simulink model "Group31_ProjectWork_EmbeddedSystem"  (R2024b)
settings: Solver=FixedStepDiscrete  StartTime=0.0  StopTime=100  FixedStep=0.1  RelTol=1e-3  EnableMultiTasking=on
libraries: stm32f4xxblockslib x6, stm32g4xxblockslib x2, stm32blockslib x2
settings Model: STM32="{\"UARTRead\":[{\"ID\":\"ProgettoEmbedded_LI_ST_gruppo33_backup_2:87\"},{\"ID\":\"ProgettoEmbedded_LI_ST_gruppo33_backup_3:87\"},{\"ID\":\"ProgettoEmbedded_LI_ST_gruppo33:87\"},{\"ID\":\"Group31_ProjectWork_EmbeddedSystem:87\"}],\"UARTWrite\":[{\"ID\":\"ProgettoEmbedded_LI_ST_gruppo33_backup_2:92\"},{\"ID\":\"ProgettoEmbedded_LI_ST_gruppo33_backup_3:92\"},{\"ID\":\"ProgettoEmbedded_LI_ST_gruppo33:92\"},{\"ID\":\"Group31_ProjectWork_EmbeddedSystem:92\"}],\"PWMOutput\":[{\"ID\":\"ProgettoEmbedded_LI_ST_gruppo33_backup_2:88\"},{\"ID\":\"ProgettoEmbedded_LI_ST_gruppo33_backup_2:104\"},{\"ID\":\"ProgettoEmbedded_LI_ST_gruppo33_backup_3:104\"},{\"ID\":\"ProgettoEmbedded_LI_ST_gruppo33_backup_3:88\"},{\"ID\":\"ProgettoEmbedded_LI_ST_gruppo33:104\"},{\"ID\":\"ProgettoEmbedded_LI_ST_gruppo33:88\"},{\"ID\":\"Group31_ProjectWork_EmbeddedSystem:104\"},{\"ID\":\"Group31_ProjectWork_EmbeddedSystem:88\"}],\"DigitalPortRead\":[{\"ID\":\"ProgettoEmbedded_LI_ST_gruppo33_backup_2:83\"},{\"ID\":\"ProgettoEmbedded_LI_ST_gruppo33_backup_2:99\"},{\"ID\":\"ProgettoEmbedded_LI_ST_gruppo33_backup_2:100\"},{\"ID\":\"ProgettoEmbedded_LI_ST_gruppo33_backup_2:101\"},{\"ID\":\"ProgettoEmbedded_LI_ST_gruppo33_backup_3:101\"},{\"ID\":\"ProgettoEmbedded_LI_ST_gruppo33_backup_3:100\"},{\"ID\":\"ProgettoEmbedded_LI_ST_gruppo33_backup_3:99\"},{\"ID\":\"ProgettoEmbedded_LI_ST_gruppo33_backup_3:83\"},{\"ID\":\"ProgettoEmbedded_LI_ST_gruppo33:101\"},{\"ID\":\"ProgettoEmbedded_LI_ST_gruppo33:100\"},{\"ID\":\"ProgettoEmbedded_LI_ST_gruppo33:99\"},{\"ID\":\"ProgettoEmbedded_LI_ST_gruppo33:83\"},{\"ID\":\"Group31_ProjectWork_EmbeddedSystem:101\"},{\"ID\":\"Group31_ProjectWork_EmbeddedSystem:100\"},{\"ID\":\"Group31_ProjectWork_EmbeddedSystem:99\"},{\"ID\":\"Group31_ProjectWork_EmbeddedSystem:83\"}],\"DigitalPortWrite\":[{\"ID\":\"ProgettoEmbedded_LI_ST_gruppo33_backup_2:93\"},{\"ID\":\"ProgettoEmbedded_LI_ST_gruppo33_backup_2:105\"},{\"ID\":\"ProgettoEmbedded_LI_ST_gruppo33_backup_3:105\"},{\"ID\":\"ProgettoEmbedded_LI_ST_gruppo33_backup_3:93\"},{\"ID\":\"ProgettoEmbedded_LI_ST_gruppo33:105\"},{\"ID\":\"ProgettoEmbedded_LI_ST_gruppo33:93\"},{\"ID\":\"Group31_ProjectWork_EmbeddedSystem:105\"},{\"ID\":\"Group31_ProjectWork_EmbeddedSystem:93\"}]}"  PacingRate=0.400000  Creator=nancy  LastModifiedBy=Alessandro
settings SolverCC: AlgebraicLoopSolver=TrustRegion  AutoInsertRateTranBlk=on
settings DataIOCC: LimitDataPoints=on
settings OptimizationCC: DefaultParameterBehavior=Inlined  EnhancedBackFolding=on  PassReuseOutputArgsAs=Individual arguments  ZeroExternalMemoryAtStartup=off  ZeroInternalMemoryAtStartup=off  MaxStackSize=512  OptimizeBlockOrder=speed  DifferentSizesBufferReuse=on  OptimizationCustomize=off  EfficientTunableParamExpr=on
settings DebuggingCC: ParameterTunabilityLossMsg=error  UnconnectedInputMsg=warning  UnconnectedOutputMsg=warning  UnconnectedLineMsg=warning  AllowSymbolicDim=off  SFUnexpectedBacktrackingDiag=warning  SFNoUnconditionalDefaultTransitionDiag=warning  SFExecutionAtInitializationDiag=none  ArithmeticOperatorsInVariantConditions=warning
settings HardwareCC: ProdBitPerPointer=32  ProdBitPerSizeT=32  ProdBitPerPtrDiffT=32  ProdLargestAtomicInteger=Long  ProdLargestAtomicFloat=Double  ProdWordSize=32  ProdLongLongMode=on  ProdHWDeviceType=ARM Compatible->ARM Cortex-M
settings ModelReferenceCC: EnableRefExpFcnMdlSchedulingChecks=on
settings SFSimCC: SimUseLocalCustomCode=off  CustomCodeUndefinedFunction=UseInterfaceOnly
settings RTWCC: Description=Embedded Coder  SystemTargetFile=ert.tlc  HardwareBoard=STM32G4xx Based  TemplateMakefile=ert_default_tmf  RTWUseLocalCustomCode=off  Toolchain=GNU Tools for ARM Embedded Processors  GPUComputeCapability=3.5  DLArmComputeVersion=19.05
settings CodeAppCC: ForceParamTrailComments=on  IgnoreCustomStorageClasses=off  OperatorAnnotations=on  SimulinkDataObjDesc=on  SFDataObjDesc=on  InsertBlockDesc=on
settings ERTTargetCC: TargetLangStandard=C99 (ISO)  CodeReplacementLibrary=ARM Cortex-M  SupportVariableSizeSignals=on  ExtModeTransport=3  ExtModeStaticAlloc=on  ExtModeStaticAllocSize=2048  ExtModeMexFile=ext_xcp  ExtModeIntrfLevel=Level2 - Open
settings ConfigComp: CovMetricSettings=dw  CovSaveCumulativeToWorkspaceVar=on  CovSaveSingleToWorkspaceVar=on  CovExternalEMLEnable=off  CovSFcnEnable=off

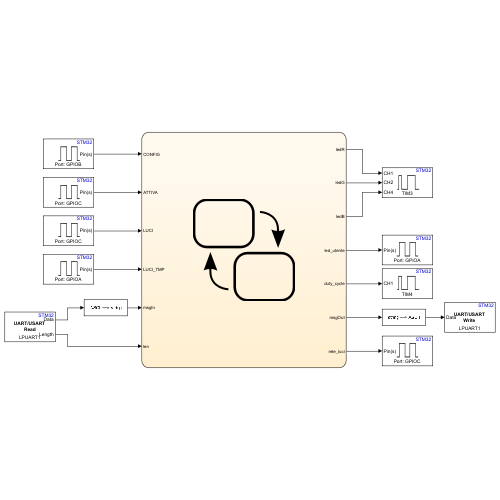
[thumbnail: Simulink's stored preview of the top-level diagram]
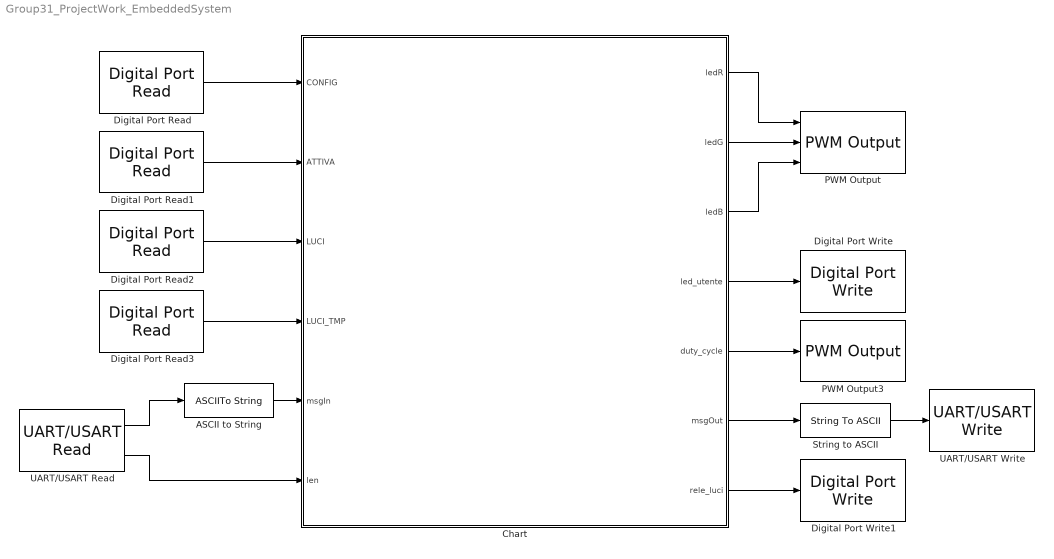
== system Group31_ProjectWork_EmbeddedSystem ==
  ASCII to String : ASCIIToString
  Chart : Stateflow chart  TreatAsAtomicUnit=on
  Digital Port Read : stm32f4xxblockslib/Digital Port Read  PortName=GPIOB  PinNumber=[0]  ReadOperation=on  IOAsArray=on  SampleTime=-1  EnableSimPort=off  hoistedMaskSrc=ECSoC/ECSimCodegen/Digital Port Read
      settings: LibrarySourceBlock=stm32g4xxblockslib/Digital Port Read
  Digital Port Read1 : stm32f4xxblockslib/Digital Port Read  PortName=GPIOC  PinNumber=[13]  ReadOperation=on  IOAsArray=on  SampleTime=-1  EnableSimPort=off  hoistedMaskSrc=ECSoC/ECSimCodegen/Digital Port Read
      settings: LibrarySourceBlock=stm32g4xxblockslib/Digital Port Read
  Digital Port Read2 : stm32f4xxblockslib/Digital Port Read  PortName=GPIOC  PinNumber=[10]  ReadOperation=on  IOAsArray=on  SampleTime=-1  EnableSimPort=off  hoistedMaskSrc=ECSoC/ECSimCodegen/Digital Port Read
      settings: LibrarySourceBlock=stm32g4xxblockslib/Digital Port Read
  Digital Port Read3 : stm32f4xxblockslib/Digital Port Read  PortName=GPIOA  PinNumber=[15]  ReadOperation=on  IOAsArray=on  SampleTime=-1  EnableSimPort=off  hoistedMaskSrc=ECSoC/ECSimCodegen/Digital Port Read
      settings: LibrarySourceBlock=stm32g4xxblockslib/Digital Port Read
  Digital Port Write : stm32f4xxblockslib/Digital Port Write  PortName=GPIOA  PinNumber=[5]  ReadOperation=off  IOAsArray=on  EnableSimPort=off  hoistedMaskSrc=ECSoC/ECSimCodegen/Digital Port Write
      settings: LibrarySourceBlock=stm32g4xxblockslib/Digital Port Write
  Digital Port Write1 : stm32f4xxblockslib/Digital Port Write  PortName=GPIOC  PinNumber=[2]  ReadOperation=off  IOAsArray=on  EnableSimPort=off  hoistedMaskSrc=ECSoC/ECSimCodegen/Digital Port Write
      settings: LibrarySourceBlock=stm32g4xxblockslib/Digital Port Write
  PWM Output : stm32g4xxblockslib/PWM Output  TimerModule=TIM3  DutycycleUnits=Percentage  EnableChannel1=on  EnableChannel2=on  EnableChannel3=off  EnableChannel4=on  EnableChannel5=off  EnableChannel6=off  EnableCounterInput=off  EnableMainOutputInput=off  EnableFrequencyInput=off  SetRCAfterCE=off  OutputDirection=off  OutputMainOutputEnableStatus=off  SampleTime=0.1  EnableSimPort=off  EnableUpdateEvent=off  EnableCaptureCompare1Event=off  EnableCaptureCompare2Event=off  EnableCaptureCompare3Event=off  EnableCaptureCompare4Event=off  EnableTriggerEvent=off  EnableBreakEvent=off  EnableBreakEvent2=off  ProcessorFamily=STM32G4  hoistedMaskSrc=ECSoC/ECSimCodegen/PWM Output
  PWM Output3 : stm32g4xxblockslib/PWM Output  TimerModule=TIM4  DutycycleUnits=Percentage  EnableChannel1=on  EnableChannel2=off  EnableChannel3=off  EnableChannel4=off  EnableChannel5=off  EnableChannel6=off  EnableCounterInput=off  EnableMainOutputInput=off  EnableFrequencyInput=off  SetRCAfterCE=off  OutputDirection=off  OutputMainOutputEnableStatus=off  SampleTime=0.1  EnableSimPort=off  EnableUpdateEvent=off  EnableCaptureCompare1Event=off  EnableCaptureCompare2Event=off  EnableCaptureCompare3Event=off  EnableCaptureCompare4Event=off  EnableTriggerEvent=off  EnableBreakEvent=off  EnableBreakEvent2=off  ProcessorFamily=STM32G4  hoistedMaskSrc=ECSoC/ECSimCodegen/PWM Output
  String to ASCII : StringToASCII  OutputVectorSize=127
  UART/USART Read : stm32blockslib/UART//USART Read  UARTModule=LPUART1  DataType=uint8  DataLength=1  BlockingMode=off  BlockingTimeout=0.1  OutputLength=on  OutputStatus=off  SampleTime=-1
      settings: LibrarySourceBlock=stm32g4xxblockslib/UART//USART Read
  UART/USART Write : stm32blockslib/UART//USART Write  UARTModule=LPUART1  LengthOfDataToSend=off  BlockingMode=off  BlockingTimeout=0.1  OutputStatus=off
      settings: LibrarySourceBlock=stm32g4xxblockslib/UART//USART Write
  wires:
  Chart/4(led_utente) -> Digital Port Write/1
  Digital Port Read/1 -> Chart/1(CONFIG)
  Chart/1(ledR) -> PWM Output/1
  Chart/6(msgOut) -> String to ASCII/1
  String to ASCII/1 -> UART/USART Write/1
  Digital Port Read1/1 -> Chart/2(ATTIVA)
  Digital Port Read2/1 -> Chart/3(LUCI)
  Digital Port Read3/1 -> Chart/4(LUCI_TMP)
  Chart/5(duty_cycle) -> PWM Output3/1
  Chart/7(rele_luci) -> Digital Port Write1/1
  Chart/2(ledG) -> PWM Output/2
  Chart/3(ledB) -> PWM Output/3
  UART/USART Read/2 -> Chart/6(len)
  UART/USART Read/1 -> ASCII to String/1
  ASCII to String/1 -> Chart/5(msgIn)

== stateflow chart Group31_ProjectWork_EmbeddedSystem/Chart ==
  state Group31_ProjectWork_EmbeddedSystem
    state INATTIVO
      en: msgOut = "Premere il pulsante ATTIVA per attivare il dispositivo" + char([13 10]) + char([13 10]);
      temperatura = 16; strTemperatura = "16";
      ledR = 0;  ledG = 0;  ledB = 255;
      led_utente = 0;
      rele_luci = 0;
      angolo = 0; strAngolo = "0";
      duty_cycle = 5;
      durata_luci = 0; strDurataLuci = "0";
      mod_luci = 0; strModLuci = "0";
      du: msgOut = "";
    state CLEAR
      en: msgOut = sprintf("\033[0;0H\033[2J");
    state ATTIVO
      state MAIN [parallel]
        settings: executionOrder=1
        state CONFIGURAZIONE
          ex:  prima_attivazione = 0;
          state CONFIGURAZIONE_COMPLETATA
            en: config_comp_init = 1;
            msgOut = char([13 10]) + fine_configurazione_iniziale();
            du: msgOut = "";
          state PRECONFIG
            en: msgOut = "";
          state INIT
            en: msgOut = initMenu();
            du: msgOut ="";
          state MENU
            en: msgOut = char([13 10]) + prepareMenu;
            du: msgOut = "";
          state setTemperatura
            en: msgOut = char([13 10]) + "TEMPERATURA: Range 16 C - 30 C" + char([13 10]);
            du: msgOut = "";
          state setVeneziane
            en: msgOut = char([13 10]) + "VENEZIANE: 0 - 9" + char([13 10]);
            du: msgOut = "";
          state setDurataLuci
            en: msgOut = char([13 10]) + "MODALITA LUCI TEMPORIZZATE: durata di accensione (5 - 30 s, 0 s: disattivata)" + char([13 10]);
            du: msgOut = "";
          state setModalitaLuci
            en: msgOut = char([13 10]) + "MODALITA LUCI: (0: spento, 1: acceso)" + char([13 10]);
            du: msgOut = "";
          state setTemperatura1
            en: uartMsg = uartMsg + msgIn;
            msgOut = msgIn; i = i + 1;
            if i == 2
            config_comp_temp = configTemperatura(uartMsg);
            end
            du: msgOut = "";
          state setVeneziane1
            en: uartMsg = uartMsg + msgIn;
            msgOut = msgIn;
            config_comp_ven = configVeneziane(uartMsg);
            du: msgOut = "";
          state setDurataLuci1
            en: uartMsg = uartMsg + msgIn;
            msgOut = msgIn; i = i + 1;
            if i > 0 && i < 3
            config_comp_durata_luci = configDurataLuci(uartMsg);
            end
            du: msgOut = "";
          state setModalitaLuci1
            en: uartMsg = uartMsg + msgIn; msgOut = msgIn;
            config_comp_mod_luci = configModLuci(uartMsg);
            du: msgOut = "";
          state ErrorDurataLuci
            en: msgOut = errorDurataLuci();
            du: msgOut = "";
          state ErrorTemperatura
            en: msgOut = errorTemperatura();
            du: msgOut = "";
          state ErrorVeneziane
            en: msgOut = errorVeneziane();
            du: msgOut = "";
          state ErrorModLuci
            en: msgOut = errorModLuci();
            du: msgOut = "";
          (default) -> PRECONFIG
          PRECONFIG -> INIT [order 2] : [prima_attivazione == 1]
          PRECONFIG -> MENU [order 1] : [prima_attivazione == 0]
          (junction 455) -> CONFIGURAZIONE_COMPLETATA [order 2] : [prima_attivazione == 1]
          (junction 455) -> MENU [order 1] : [prima_attivazione == 0]
          MENU -> setModalitaLuci [order 1] : [len > 0 && msgIn == "1"]
          MENU -> setVeneziane [order 3] : [len > 0 && msgIn == "4"]
          (junction 529) -> MENU [order 2] : {prima_attivazione == 0}
          (junction 430) -> MENU [order 1] : [prima_attivazione == 0]
          MENU -> setDurataLuci [order 4] : [len > 0 && msgIn == "2"]
          (junction 427) -> MENU [order 1] : [prima_attivazione == 0]
          MENU -> setTemperatura [order 2] : [len > 0 && msgIn == "3"]
          INIT -> setModalitaLuci : after(3,sec)
          (junction 529) -> setDurataLuci [order 1] : [prima_attivazione == 1]
          (junction 430) -> setVeneziane [order 2] : [prima_attivazione == 1]
          setVeneziane1 -> (junction 455) [order 1] : [config_comp_ven == 1 && len > 0 && msgIn == char(13)]{angolo = applyConv(uartMsg); strAngolo = uartMsg;}
          setVeneziane -> setVeneziane1 : [len >0]{uartMsg="";}
          ErrorVeneziane -> setVeneziane : [len > 0 && msgIn == char(13)]
          setDurataLuci -> setDurataLuci1 : [len >0]{uartMsg=""; i = 0;}
          ErrorDurataLuci -> setDurataLuci : [len > 0 && msgIn == char(13)]
          setModalitaLuci -> setModalitaLuci1 : [len > 0]{uartMsg="";}
          ErrorModLuci -> setModalitaLuci : [len > 0 && msgIn == char(13)]
          (junction 427) -> setTemperatura [order 2] : [prima_attivazione == 1]
          setTemperatura -> setTemperatura1 : [len >0]{uartMsg=""; i = 1;}
          ErrorTemperatura -> setTemperatura : [len > 0 && msgIn == char(13)]
          setModalitaLuci1 -> (junction 529) [order 1] : [config_comp_mod_luci == 1 && len > 0 && msgIn == char(13)]{mod_luci = applyConv(uartMsg); strModLuci = uartMsg;}
          setDurataLuci1 -> (junction 427) [order 1] : [config_comp_durata_luci == 1 && len > 0 && msgIn == char(13)]{durata_luci = applyConv(uartMsg); strDurataLuci = uartMsg;}
          setTemperatura1 -> (junction 430) [order 2] : [config_comp_temp == 1 && len > 0 && msgIn == char(13)]{temperatura = applyConv(uartMsg); strTemperatura = uartMsg;}
          setDurataLuci1 -> setDurataLuci1 [order 3] : [rising(len)]
          setTemperatura1 -> setTemperatura1 [order 3] : [rising(len)]
          setModalitaLuci1 -> ErrorModLuci [order 2] : [config_comp_mod_luci == 0 && len > 0 && msgIn == char(13)]
          setDurataLuci1 -> ErrorDurataLuci [order 2] : [config_comp_durata_luci == 0 && len > 0 && msgIn == char(13)]
          setTemperatura1 -> ErrorTemperatura [order 1] : [config_comp_temp == 0 && len > 0 && msgIn == char(13)]
          setVeneziane1 -> ErrorVeneziane [order 2] : [config_comp_ven == 0 && len > 0 && msgIn == char(13)]
        state OPERAZIONE
          state NOTIFICA_STATO [parallel]
            settings: executionOrder=2
            state NOT2
              en: %% VENEZIANE
              if angolo == 0
              printVen = "CHIUSE";
              elseif angolo == 9
              printVen = "APERTE";
              else
              printVen = "APERTE PARZIALMENTE con Preset " + strAngolo;
              end
              %% LUCI
              if rele_luci == 1 || mod_luci == 1
              printLuci = "ACCESE";
              else
              printLuci = "SPENTE";
              end
              msgOut =  char([13 10]) + notifica(strTemperatura, printVen, printLuci) + char([13 10]);
              du: msgOut = "";
            (default) -> NOT2
            NOT2 -> NOT2 : after(10, sec)
          state LUCI [parallel]
            settings: executionOrder=3
            state LUCI_SPENTE
              en: rele_luci = 0;
              mod_luci = 0;
            state LUCI_TEMPORIZZATE
              en: rele_luci = 1;
            state LUCI_ACCESE
              en: rele_luci = 1;
            (default) -> LUCI_SPENTE [order 2]
            LUCI_SPENTE -> LUCI_TEMPORIZZATE [order 2] : [rising(LUCI_TMP) && durata_luci > 0]
            LUCI_TEMPORIZZATE -> LUCI_SPENTE : [rising(LUCI) || after(durata_luci,sec)]
            LUCI_ACCESE -> LUCI_SPENTE [order 2] : [rising(LUCI)]
            LUCI_SPENTE -> LUCI_ACCESE [order 1] : [rising(LUCI)]
            LUCI_ACCESE -> LUCI_TEMPORIZZATE [order 1] : [rising(LUCI_TMP) && durata_luci > 0]
            (default) -> LUCI_ACCESE [order 1] : [mod_luci == 1]
          state TEMPERATURA [parallel]
            en: [ledR, ledG, ledB] = opTemperatura(temperatura);
            settings: executionOrder=1
          state VENEZIANE [parallel]
            en: duty_cycle = opVeneziane(angolo);
            settings: executionOrder=4
        (default) -> CONFIGURAZIONE
        CONFIGURAZIONE -> OPERAZIONE : [rising(CONFIG) && config_comp_init == 1]
        OPERAZIONE -> CONFIGURAZIONE : [rising(CONFIG)]
      state LED_UTENTE [parallel]
        settings: executionOrder=2
        state SPENTO
          en: led_utente = 0;
        state ACCESO
          en: led_utente=1;
        (default) -> SPENTO
        SPENTO -> ACCESO : [after(0.5,sec)]
        ACCESO -> SPENTO : [after(0.5,sec)]
    (default) -> CLEAR
    CLEAR -> INATTIVO
    INATTIVO -> ATTIVO : [rising(ATTIVA)]
    ATTIVO -> INATTIVO : [rising(ATTIVA) && config_comp_init == 1]
  (default) -> Group31_ProjectWork_EmbeddedSystem : {prima_attivazione = 1;}
  data: str function_input; val function_output; msg function_output; msgOut function_output; msgOut function_output; msg function_output; msg function_output; msg function_output; msg function_output; msg function_input; valModLuci function_output; msg function_input; valDurataLuci function_output; msg function_input; valTemp function_output; msg function_input; valAngle function_output; newChar function_input; newVal function_output; msg function_output; printTemp function_input; printVen function_input; printLuci function_input; temperatura function_input; ledR function_output; ledG function_output; ledB function_output; angolo function_input; duty_cycle function_output; CONFIG input size=1; ATTIVA input size=1; LUCI input size=1; LUCI_TMP input size=1; ledR output size=1 =0; ledG output size=1 =0; ledB output size=1 =255; led_utente output size=1 =0; duty_cycle output size=1 =5; temperatura local =16; durata_luci local =0; angolo local =0; prima_attivazione local double =1; msgIn input string; msgOut output string; rele_luci output size=1 =0; mod_luci local double size=1 =0; len input size=1; uartMsg local string; config_comp_mod_luci local; config_comp_durata_luci local; config_comp_temp local; config_comp_ven local; i local; strTemperatura local; strDurataLuci local; strAngolo local; strModLuci local; config_comp_init local =0; printVen local; printLuci local
  function val  = myStr2Double(str):
    | function val = myStr2Double(str)
    |     % Verifica input valido (solo cifre)
    |     if isempty(str)
    |         error('Stringa vuota.');
    |     end
    |  
    |     n = length(str);
    |     val = 0;
    |  
    |     for i = 1:n
    |         c = str(i);
    |         % Controllo che sia una cifra
    |         if c < '0' || c > '9'
    |             error('Carattere non numerico nella stringa: "%s"', c);
    |         end
    |         % Converti il carattere in cifra numerica (codice ASCII)
    |         digit = double(c) - double('0');
    |         val = real(val * 10 + digit);
    |     end
    | end
  function msg = fine_configurazione_iniziale:
    | function msg = fine_configurazione_iniziale
    |     CLRF = char([13 10]);
    |     msg = CLRF + "Configurazione iniziale completata." + CLRF + ...
    |           "Per entrare nella modalita operativa, premere il pulsante CONFIG.";
    | end
  function msgOut = initMenu:
    | function msgOut = initMenu()
    |     CLRF = char([13 10]);
    | 
    |     msgOut = "Benvenuto nell ambiente domotico!" + CLRF + ...
    |           "Alla prima attivazione, e necessario configurare tutte le funzionalita" + CLRF;
    | 
    | end
  function msgOut = prepareMenu:
    | function msgOut = prepareMenu
    |     CLRF = char([13 10]);
    |     
    |     msgOut = CLRF + "==== MENU ====" + CLRF + ...
    |         "1. Luci ON/OFF" + CLRF + ...
    |         "2. Luci Temporizzate" + CLRF + ...
    |         "3. Temperatura" + CLRF + ...
    |         "4. Veneziane" + CLRF + ...
    |         "Premi CONFIG" + CLRF;
    | end
  function msg = errorDurataLuci:
    | function msg = errorDurataLuci()
    |     CLRF = char([13 10]);
    |     msg = CLRF + "Valore DURATA LUCI non valido." + CLRF + ...
    |         "Premi INVIO per reinserirlo" + CLRF;
    | end
  function msg = errorTemperatura:
    | function msg = errorTemperatura()
    |     CLRF = char([13 10]);
    |     msg = CLRF + "Valore TEMPERATURA non valido." + CLRF + ...
    |         "Premi INVIO per reinserirlo" + CLRF;
    | end
  function msg = errorVeneziane:
    | function msg = errorVeneziane
    |     CLRF = char([13 10]);
    |     msg = CLRF + "Valore VENEZIANE non valido." + CLRF + ...
    |         "Premi INVIO per reinserirlo" + CLRF;
    | end
  function msg = errorModLuci:
    | function msg = errorModLuci()
    |     CLRF = char([13 10]);
    |     msg = CLRF + "Valore MODALITA LUCI non valido." + CLRF + ...
    |         "Premi INVIO per reinserirlo" + CLRF;
    | end
  function valModLuci = configModLuci(msg):
    | function valModLuci = configModLuci(msg)
    |     numLights = myStr2Double(char(msg));
    |     valModLuci = 0;
    |     
    |     if numLights == 1 || numLights == 0
    |        valModLuci = 1; 
    |     end
    | end
  function valDurataLuci  = configDurataLuci(msg):
    | function valDurataLuci  = configDurataLuci(msg)
    |     numDurataLuci = myStr2Double(char(msg));
    |     valDurataLuci = 0;
    |     
    |     if numDurataLuci > 4 && numDurataLuci < 31 || numDurataLuci == 0
    |        valDurataLuci = 1; 
    |     end
    | end
  function valTemp  = configTemperatura(msg):
    | function valTemp  = configTemperatura(msg)
    |     numTemp = myStr2Double(char(msg));
    |     valTemp = 0;
    |     
    |     if numTemp > 15 && numTemp < 31
    |        valTemp = 1; 
    |     end
    | end
  function valAngle  = configVeneziane(msg):
    | function valAngle  = configVeneziane(msg)
    |     numPreset = myStr2Double(char(msg));
    |     valAngle = 0;
    |     
    |     if numPreset >= 0 && numPreset < 10
    |        valAngle = 1; 
    |     end
    | end
  function newVal = applyConv(newChar):
    | function newVal = applyConv(newChar)
    |     newVal = myStr2Double(char(newChar));
    | end
  function msg = notifica(printTemp, printVen, printLuci):
    | function msg = notifica(printTemp, printVen, printLuci)
    |     CLRF = char([13 10]);
    | 
    |     %% STAMPA NOTIFICA
    |     msg = CLRF + "=== STATUS ===" + CLRF + ...
    |         "Temperatura: " + printTemp + " C" + CLRF + ...
    |         "Veneziane: " + printVen + CLRF + ...
    |         "Luci: " + printLuci;
    | end
  function [ledR, ledG, ledB] = opTemperatura(temperatura):
    | function [ledR, ledG, ledB] = opTemperatura(temperatura)
    |     % BLU
    |     if temperatura >= 16 && temperatura <= 18
    |         ledR = 0;
    |         ledG = 0;
    |         ledB = 255;
    |     % VIOLA
    |     elseif temperatura >= 19 && temperatura <= 21
    |         ledR = 127;
    |         ledG = 0;
    |         ledB = 255;
    |     % GIALLO
    |     elseif temperatura >= 22 && temperatura <= 24
    |         ledR = 255;
    |         ledG = 255;
    |         ledB = 0;
    |     % ARANCIONE
    |     elseif temperatura >= 25 && temperatura <= 27
    |         ledR = 255;
    |         ledG = 127;
    |         ledB = 0;
    |     % ROSSO
    |     elseif temperatura >= 28 && temperatura <= 30
    |         ledR = 255;
    |         ledG = 0;
    |         ledB = 0;
    |     % FALLBACK
    |     else
    |         ledR = 0;
    |         ledG = 0;
    |         ledB = 255;
    |     end
    |     
    | end
  function duty_cycle = opVeneziane(angolo):
    | function duty_cycle = opVeneziane(angolo)
    |     duty_min = 5;    % 5% = 0°
    |     duty_max = 10;    % 10% = 180°
    |     angolo = angolo*20;
    | 
    |     if angolo >= 0 && angolo <= 180
    |         duty_cycle = duty_min + (angolo / 180) * (duty_max - duty_min);
    |     else
    |         duty_cycle = 0;  
    |     end
    | end
